simulink model "zn1_template"  (R2015a)
settings: Solver=ode1  SolverMode=SingleTasking  StartTime=0.0  StopTime=10  FixedStep=0.01  RelTol=1e-3
values from neighbouring files (symbols this model uses):
  KP = 0.6*Ku    (= 6.62800387681)    [exp9.m]    (also in exp9_ptestes.m = 2.42800387681)
  N = 10    [exp9.m]    (also in exp9_ptestes.m)
  Td = Tu/8    (= 0.0875)    [exp9.m]    (also in exp9_ptestes.m = 0.1275)
  Ti = Tu/2    (= 0.35)    [exp9.m]    (also in exp9_ptestes.m = 0.5)
settings Model: CovSFcnEnable=off  Creator=rpm  LastModifiedBy=Caio
settings DataIOCC: LimitDataPoints=off  SignalLoggingSaveFormat=ModelDataLogs  SaveOutput=off  SignalLogging=off  TimeSaveName=t
settings OptimizationCC: ExpressionDepthLimit=2147483647  InitFltsAndDblsToZero=on
settings DebuggingCC: UnderspecifiedInitializationDetection=Classic  MergeDetectMultiDrivingBlocksExec=none  FcnCallInpInsideContextMsg=UseLocalSettings  StateNameClashWarn=warning
settings GRTTargetCC: CombineOutputUpdateFcns=off  GRTInterface=on

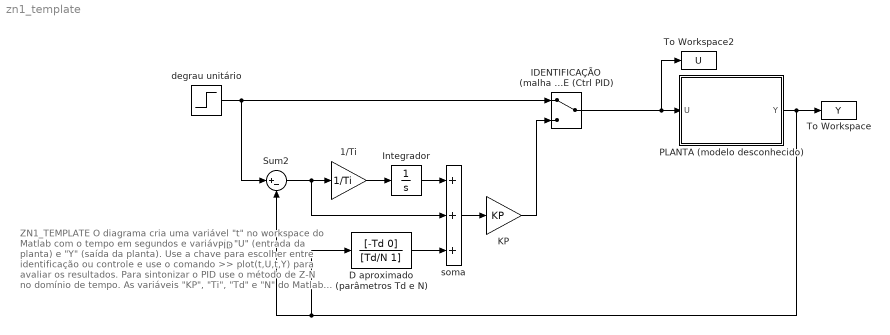
== system zn1_template ==
  note: ZN1_TEMPLATE
      |
      | O diagrama cria uma variável "t" no workspace
      | do Matlab com o tempo em segundos e variáveis
      | "U" (entrada da planta) e "Y" (saída da planta).
      |
      | Use a chave para escolher entre identificação
      | ou controle e use o comando
      |
      | >> plot(t,U,t,Y)
      |
      | para avaliar os resultados.
      |
      | Para sintonizar o PID use o método de Z-N
      | no domínio de tempo.
      |
      | As variáveis "KP", "Ti", "Td" e "N" do Matlab
      | contêm a sintonia do controlador.
      | (é necessário criá-las para que não haja
      | erros na simulação, mesmo se não
      | forem usadas).
      |
      | IMPORTANTE: Não há garantias de que o método
      | seja capaz de produzir um bom desempenho ou
      | mesmo que funcione.
  note: PID
  1/Ti : Gain  Gain=1/Ti
  D aproximado (parâmetros Td e N) : TransferFcn  Numerator=[-Td 0]  Denominator=[Td/N 1]
  IDENTIFICAÇÃO (malha aberta) ou CONTROLE (Ctrl PID) : ManualSwitch
  Integrador : Integrator
  KP : Gain  Gain=KP
  PLANTA (modelo desconhecido) : Subsystem
  Sum2 : Sum  Inputs=|+-
  To Workspace : ToWorkspace  VariableName=Y  SampleTime=-1
  To Workspace2 : ToWorkspace  VariableName=U  SampleTime=-1
  degrau unitário : Step  Time=0  SampleTime=0
  soma : Sum  Inputs=+++
  wires:
  IDENTIFICAÇÃO (malha aberta) ou CONTROLE (Ctrl PID)/1 -> To Workspace2/1, PLANTA (modelo desconhecido)/1(U)
  degrau unitário/1 -> IDENTIFICAÇÃO (malha aberta) ou CONTROLE (Ctrl PID)/1, Sum2/1
  KP/1 -> IDENTIFICAÇÃO (malha aberta) ou CONTROLE (Ctrl PID)/2
  soma/1 -> KP/1
  1/Ti/1 -> Integrador/1
  Sum2/1 -> 1/Ti/1, soma/2
  PLANTA (modelo desconhecido)/1(Y) -> To Workspace/1, Sum2/2, D aproximado (parâmetros Td e N)/1
  Integrador/1 -> soma/1
  D aproximado (parâmetros Td e N)/1 -> soma/3

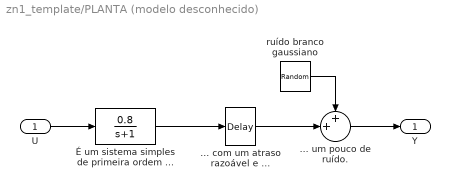
== system zn1_template/PLANTA (modelo desconhecido) ==
  U : Inport
  ... com um atraso razoável e ... : TransportDelay
  ... um pouco de ruído. : Sum  Inputs=++|
  ruído branco gaussiano : RandomNumber  Variance=0.0001  SampleTime=0
  É um sistema simples de primeira ordem ... : TransferFcn  Numerator=[0.8]  Denominator=[1 1]
  Y : Outport
  wires:
  É um sistema simples de primeira ordem .../1 -> ... com um atraso razoável e .../1
  U/1 -> É um sistema simples de primeira ordem .../1
  ... com um atraso razoável e .../1 -> ... um pouco de ruído./2
  ... um pouco de ruído./1 -> Y/1
  ruído branco gaussiano/1 -> ... um pouco de ruído./1
